simulink model "modified_splitter_IEcontrol"  (R2020a)
settings: Solver=VariableStepAuto  StartTime=0.0  StopTime=10.0  RelTol=1e-3
model workspace (MATLAB code in the model file):
  | v_M_exhale = 490; % cmH2O (PEEP)
  | v_M_inhale = 1471; % (PIP)
  | R_M = 0; %
  | 
  | R_V1 = 5670; % cmH2O/L/s
  | R_V2 = 5670;
  | R_I1 = 5670; % tube length = 1.8 ms
  | R_I2 = 5670;
  | R_EV1 = 0;
  | R_EV2 = 0;
  | 
  | R_L1 = 196133;
  | R_L2 = 196133;
  | C_L1 = 5.50647e-7; % L/cmH2O
  | C_L2 = 5.50647e-7;
  | R_ETT1 = 784000;
  | R_ETT2 = 784000;
  | 
  | % === artificial patients (bags)s ====
  | R_aL1 = 196133;
  | R_aL2 = 196133;
  | C_aL1 = 5.50647e-7;
  | C_aL2 = 5.50647e-7;
  | % =======
  | 
  | R_E1 = 5670;
  | R_E2 = 5670;
  | R_O = 0;
  | 
  | RR = 15;
  | I = 1;
  | E = 2;
  | IE_ratio = I/ E;
libraries: fl_lib x37, nesl_utility x14
settings Model: Creator=jsolislemus  LastModifiedBy=jsolislemus

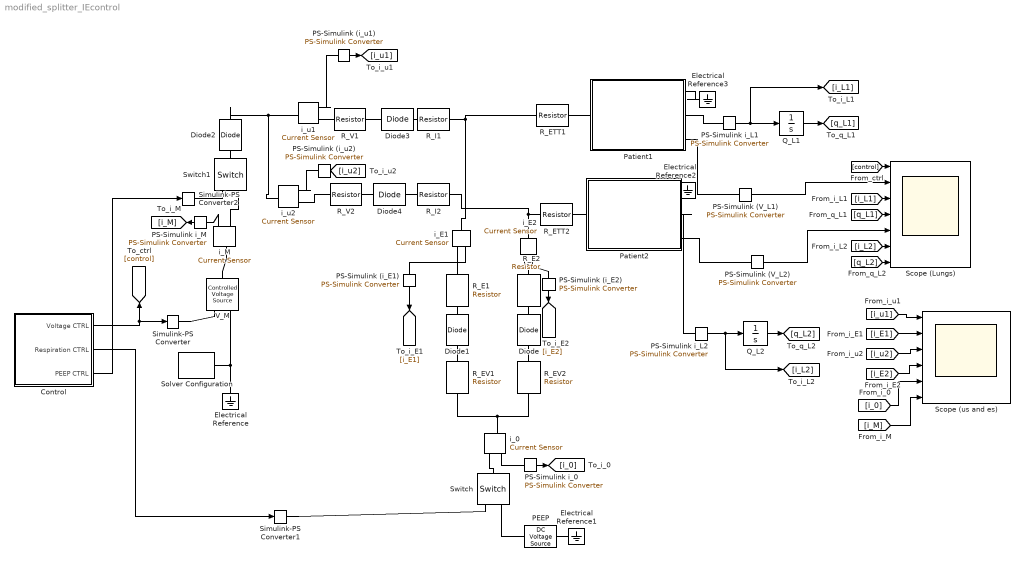
== system modified_splitter_IEcontrol ==
  Control : Subsystem
  Diode{,1..4} (5 alike) : fl_lib/Electrical/Electrical Elements/Diode  Vf=0.6 V  Ron=0.3 Ohm  Goff=1e-8 1/Ohm  i_specify=off  i_priority=None  i=0 A  i_nominal_specify=off  i_nominal_unit=A  i_nominal_value=1  v_specify=off  v_priority=None  v=0 V  v_nominal_specify=off  v_nominal_unit=V  v_nominal_value=1
  Electrical Reference{,1..3} (4 alike) : fl_lib/Electrical/Electrical Elements/Electrical Reference
  PEEP : fl_lib/Electrical/Electrical Sources/DC Voltage Source  v0=v_M_exhale V
  PS-Simulink (V_L1) : nesl_utility/PS-Simulink Converter  PhysicalDomain=network_engine_domain  SubClassName=ps_output  LeftPortType=input  RightPortType=output  PseudoPeriodic=off  Frequencies=[]  Unit=inherit  AffineConversion=off
  PS-Simulink (V_L2) : nesl_utility/PS-Simulink Converter  PhysicalDomain=network_engine_domain  SubClassName=ps_output  LeftPortType=input  RightPortType=output  PseudoPeriodic=off  Frequencies=[]  Unit=inherit  AffineConversion=off
  PS-Simulink (i_E1) : nesl_utility/PS-Simulink Converter  PhysicalDomain=network_engine_domain  SubClassName=ps_output  LeftPortType=input  RightPortType=output  PseudoPeriodic=off  Frequencies=[]  Unit=inherit  AffineConversion=off
  PS-Simulink (i_E2) : nesl_utility/PS-Simulink Converter  PhysicalDomain=network_engine_domain  SubClassName=ps_output  LeftPortType=input  RightPortType=output  PseudoPeriodic=off  Frequencies=[]  Unit=inherit  AffineConversion=off
  PS-Simulink (i_u1) : nesl_utility/PS-Simulink Converter  PhysicalDomain=network_engine_domain  SubClassName=ps_output  LeftPortType=input  RightPortType=output  PseudoPeriodic=off  Frequencies=[]  Unit=inherit  AffineConversion=off
  PS-Simulink (i_u2) : nesl_utility/PS-Simulink Converter  PhysicalDomain=network_engine_domain  SubClassName=ps_output  LeftPortType=input  RightPortType=output  PseudoPeriodic=off  Frequencies=[]  Unit=inherit  AffineConversion=off
  PS-Simulink i_0 : nesl_utility/PS-Simulink Converter  PhysicalDomain=network_engine_domain  SubClassName=ps_output  LeftPortType=input  RightPortType=output  PseudoPeriodic=off  Frequencies=[]  Unit=inherit  AffineConversion=off
  PS-Simulink i_L1 : nesl_utility/PS-Simulink Converter  PhysicalDomain=network_engine_domain  SubClassName=ps_output  LeftPortType=input  RightPortType=output  PseudoPeriodic=off  Frequencies=[]  Unit=inherit  AffineConversion=off
  PS-Simulink i_L2 : nesl_utility/PS-Simulink Converter  PhysicalDomain=network_engine_domain  SubClassName=ps_output  LeftPortType=input  RightPortType=output  PseudoPeriodic=off  Frequencies=[]  Unit=inherit  AffineConversion=off
  PS-Simulink i_M : nesl_utility/PS-Simulink Converter  PhysicalDomain=network_engine_domain  SubClassName=ps_output  LeftPortType=input  RightPortType=output  PseudoPeriodic=off  Frequencies=[]  Unit=inherit  AffineConversion=off
  Patient1 : Subsystem
  Patient2 : Subsystem
  Q_L1 : Integrator
  Q_L2 : Integrator
  R_E1 : fl_lib/Electrical/Electrical Elements/Resistor  R=R_E1 Ohm  i_specify=off  i_priority=None  i=0 A  i_nominal_specify=off  i_nominal_unit=A  i_nominal_value=1  v_specify=off  v_priority=None  v=0 V  v_nominal_specify=off  v_nominal_unit=V  v_nominal_value=1
  R_E2 : fl_lib/Electrical/Electrical Elements/Resistor  R=R_E2 Ohm  i_specify=off  i_priority=None  i=0 A  i_nominal_specify=off  i_nominal_unit=A  i_nominal_value=1  v_specify=off  v_priority=None  v=0 V  v_nominal_specify=off  v_nominal_unit=V  v_nominal_value=1
  R_ETT1 : fl_lib/Electrical/Electrical Elements/Resistor  R=R_ETT1 Ohm  i_specify=off  i_priority=None  i=0 A  i_nominal_specify=off  i_nominal_unit=A  i_nominal_value=1  v_specify=off  v_priority=None  v=0 V  v_nominal_specify=off  v_nominal_unit=V  v_nominal_value=1
  R_ETT2 : fl_lib/Electrical/Electrical Elements/Resistor  R=R_ETT2 Ohm  i_specify=off  i_priority=None  i=0 A  i_nominal_specify=off  i_nominal_unit=A  i_nominal_value=1  v_specify=off  v_priority=None  v=0 V  v_nominal_specify=off  v_nominal_unit=V  v_nominal_value=1
  R_EV1 : fl_lib/Electrical/Electrical Elements/Resistor  R=R_EV1 Ohm  i_specify=off  i_priority=None  i=0 A  i_nominal_specify=off  i_nominal_unit=A  i_nominal_value=1  v_specify=off  v_priority=None  v=0 V  v_nominal_specify=off  v_nominal_unit=V  v_nominal_value=1
  R_EV2 : fl_lib/Electrical/Electrical Elements/Resistor  R=R_EV2 Ohm  i_specify=off  i_priority=None  i=0 A  i_nominal_specify=off  i_nominal_unit=A  i_nominal_value=1  v_specify=off  v_priority=None  v=0 V  v_nominal_specify=off  v_nominal_unit=V  v_nominal_value=1
  R_I1 : fl_lib/Electrical/Electrical Elements/Resistor  R=R_I1 Ohm  i_specify=off  i_priority=None  i=0 A  i_nominal_specify=off  i_nominal_unit=A  i_nominal_value=1  v_specify=off  v_priority=None  v=0 V  v_nominal_specify=off  v_nominal_unit=V  v_nominal_value=1
  R_I2 : fl_lib/Electrical/Electrical Elements/Resistor  R=R_I2 Ohm  i_specify=off  i_priority=None  i=0 A  i_nominal_specify=off  i_nominal_unit=A  i_nominal_value=1  v_specify=off  v_priority=None  v=0 V  v_nominal_specify=off  v_nominal_unit=V  v_nominal_value=1
  R_V1 : fl_lib/Electrical/Electrical Elements/Resistor  R=R_V1 Ohm  i_specify=off  i_priority=None  i=0 A  i_nominal_specify=off  i_nominal_unit=A  i_nominal_value=1  v_specify=off  v_priority=None  v=0 V  v_nominal_specify=off  v_nominal_unit=V  v_nominal_value=1
  R_V2 : fl_lib/Electrical/Electrical Elements/Resistor  R=R_V2 Ohm  i_specify=off  i_priority=None  i=0 A  i_nominal_specify=off  i_nominal_unit=A  i_nominal_value=1  v_specify=off  v_priority=None  v=0 V  v_nominal_specify=off  v_nominal_unit=V  v_nominal_value=1
  Scope (Lungs) : Scope  NumInputPorts=7
  Scope (us and es) : Scope  NumInputPorts=6
  Simulink-PS Converter : nesl_utility/Simulink-PS Converter  PhysicalDomain=network_engine_domain  SubClassName=ps_input  LeftPortType=input  RightPortType=output  PseudoPeriodic=off  Frequencies=[]  NoiseDistribution=none  NoiseParameters=[]  Unit=1  AffineConversion=off  FilteringAndDerivatives=provide  SimscapeFilterOrder=1  InputFilterTimeConstant=0.001  UdotUserProvided=0
  Simulink-PS Converter1 : nesl_utility/Simulink-PS Converter  PhysicalDomain=network_engine_domain  SubClassName=ps_input  LeftPortType=input  RightPortType=output  PseudoPeriodic=off  Frequencies=[]  NoiseDistribution=none  NoiseParameters=[]  Unit=1  AffineConversion=off  FilteringAndDerivatives=provide  SimscapeFilterOrder=1  InputFilterTimeConstant=0.001  UdotUserProvided=0
  Simulink-PS Converter2 : nesl_utility/Simulink-PS Converter  PhysicalDomain=network_engine_domain  SubClassName=ps_input  LeftPortType=input  RightPortType=output  PseudoPeriodic=off  Frequencies=[]  NoiseDistribution=none  NoiseParameters=[]  Unit=1  AffineConversion=off  FilteringAndDerivatives=provide  SimscapeFilterOrder=1  InputFilterTimeConstant=0.001  UdotUserProvided=0
  Solver Configuration : nesl_utility/Solver Configuration  PhysicalDomain=network_engine_domain  SubClassName=solver  LeftPortType=input  RightPortType=generic  Tones=[]  Harmonics=[]  SimulateNoise=off  Profile=off  UseLocalSampling=off  EnableSwitchedLinearOptims=on  FrequencyDomain=off  UseCCode=off  RelTol=0.001  AbsTol=1e-06  MinStep=1e-09  ToWorkspace=off  RevertToSquareIcSolve=off  NumHomotopyIterations=100  PhasorMode=off  PhasorModeNumHarmonics=1  DoDC=off  ResidualTolerance=1e-09  UseLocalSolver=off  LocalSolverChoice=NE_BACKWARD_EULER_ADVANCER  LocalSolverSampleTime=0.001  DoFixedCost=off  MaxNonlinIter=3  MaxModeIter=2  LinearAlgebra=auto  EquationFormulation=NE_TIME_EF  DelaysMemoryBudget=1024  AutomaticFiltering=on  FilteringTimeConstant=0.001  PartitionStorageMethod=AS_NEEDED  PartitionMemoryBudget=1024  PartitionMethod=ROBUST
  Switch : fl_lib/Electrical/Electrical Elements/Switch  R_closed=0.01 Ohm  G_open=1e-8 1/Ohm  Threshold=0.5  i_specify=off  i_priority=None  i=0 A  i_nominal_specify=off  i_nominal_unit=A  i_nominal_value=1  v_specify=off  v_priority=None  v=0 V  v_nominal_specify=off  v_nominal_unit=V  v_nominal_value=1
  Switch1 : fl_lib/Electrical/Electrical Elements/Switch  R_closed=0.01 Ohm  G_open=1e-8 1/Ohm  Threshold=0.5  i_specify=off  i_priority=None  i=0 A  i_nominal_specify=off  i_nominal_unit=A  i_nominal_value=1  v_specify=off  v_priority=None  v=0 V  v_nominal_specify=off  v_nominal_unit=V  v_nominal_value=1
  V_M : fl_lib/Electrical/Electrical Sources/Controlled Voltage Source
  i_0 : fl_lib/Electrical/Electrical Sensors/Current Sensor
  i_E1 : fl_lib/Electrical/Electrical Sensors/Current Sensor
  i_E2 : fl_lib/Electrical/Electrical Sensors/Current Sensor
  i_M : fl_lib/Electrical/Electrical Sensors/Current Sensor
  i_u1 : fl_lib/Electrical/Electrical Sensors/Current Sensor
  i_u2 : fl_lib/Electrical/Electrical Sensors/Current Sensor
  wires:
  PS-Simulink i_L1/1 -> [i_L1], Q_L1/1
  PS-Simulink i_L2/1 -> [i_L2], Q_L2/1
  Q_L1/1 -> [q_L1]
  Q_L2/1 -> [q_L2]
  PS-Simulink (i_u1)/1 -> [i_u1]
  [i_u1] -> Scope (us and es)/1
  [i_u2] -> Scope (us and es)/3
  PS-Simulink (i_u2)/1 -> [i_u2]
  [i_E1] -> Scope (us and es)/2
  [i_E2] -> Scope (us and es)/4
  PS-Simulink (i_E2)/1 -> [i_E2]
  [i_0] -> Scope (us and es)/5
  PS-Simulink i_0/1 -> [i_0]
  PS-Simulink i_M/1 -> [i_M]
  [i_M] -> Scope (us and es)/6
  PS-Simulink (i_E1)/1 -> [i_E1]
  [control] -> Scope (Lungs)/1
  [q_L2] -> Scope (Lungs)/7
  [i_L2] -> Scope (Lungs)/6
  [q_L1] -> Scope (Lungs)/4
  PS-Simulink (V_L1)/1 -> Scope (Lungs)/2
  PS-Simulink (V_L2)/1 -> Scope (Lungs)/5
  [i_L1] -> Scope (Lungs)/3
  Control/1(Voltage CTRL) -> [control], Simulink-PS Converter/1
  Control/2(Respiration CTRL) -> Simulink-PS Converter1/1
  Control/3(PEEP CTRL) -> Simulink-PS Converter2/1
  connections:
  Simulink-PS Converter/RConn1 -- V_M/RConn1
  V_M/RConn2 -- Solver Configuration/RConn1 -- Electrical Reference/LConn1
  i_u1/LConn1 -- Diode2/RConn1 -- i_u2/LConn1
  R_ETT2/LConn1 -- R_I2/RConn1 -- i_E2/LConn1
  Simulink-PS Converter1/RConn1 -- Switch/RConn1
  i_u1/RConn2 -- R_V1/LConn1
  i_u2/RConn2 -- R_V2/LConn1
  i_E2/RConn2 -- R_E2/LConn1
  i_M/LConn1 -- V_M/LConn1
  i_0/RConn2 -- Switch/LConn1
  i_u1/RConn1 -- PS-Simulink (i_u1)/LConn1
  i_u2/RConn1 -- PS-Simulink (i_u2)/LConn1
  i_0/RConn1 -- PS-Simulink i_0/LConn1
  i_E2/RConn1 -- PS-Simulink (i_E2)/LConn1
  i_E1/RConn1 -- PS-Simulink (i_E1)/LConn1
  i_M/RConn1 -- PS-Simulink i_M/LConn1
  Electrical Reference3/LConn1 -- Patient1/RConn1
  Patient1/RConn2 -- PS-Simulink i_L1/LConn1
  Patient1/RConn3 -- PS-Simulink (V_L1)/LConn1
  Electrical Reference2/LConn1 -- Patient2/RConn1
  Patient2/RConn3 -- PS-Simulink (V_L2)/LConn1
  Patient2/RConn2 -- PS-Simulink i_L2/LConn1
  R_E1/LConn1 -- i_E1/RConn2
  R_ETT1/RConn1 -- Patient1/LConn1
  R_ETT1/LConn1 -- i_E1/LConn1 -- R_I1/RConn1
  R_ETT2/RConn1 -- Patient2/LConn1
  Diode/LConn1 -- R_E2/RConn1
  Switch1/LConn1 -- Diode2/LConn1
  Switch1/RConn2 -- i_M/RConn2
  Simulink-PS Converter2/RConn1 -- Switch1/RConn1
  PEEP/RConn1 -- Electrical Reference1/LConn1
  Switch/RConn2 -- PEEP/LConn1
  Diode1/LConn1 -- R_E1/RConn1
  Diode3/LConn1 -- R_V1/RConn1
  Diode3/RConn1 -- R_I1/LConn1
  Diode4/LConn1 -- R_V2/RConn1
  Diode4/RConn1 -- R_I2/LConn1
  R_EV1/LConn1 -- Diode1/RConn1
  R_EV2/LConn1 -- Diode/RConn1
  R_EV1/RConn1 -- R_EV2/RConn1 -- i_0/LConn1

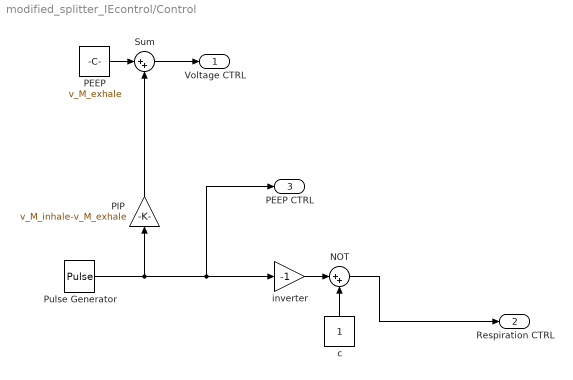
== system modified_splitter_IEcontrol/Control ==
  NOT : Sum  Inputs=|++
  PEEP : Constant  Value=v_M_exhale
  PIP : Gain  Gain=v_M_inhale-v_M_exhale
  Pulse Generator : DiscretePulseGenerator  PulseType=Time based  Period=60 / RR  PulseWidth=IE_ratio/(IE_ratio+1)*100
  Sum : Sum  Inputs=|++
  c : Constant
  inverter : Gain  Gain=-1
  Voltage CTRL : Outport
  Respiration CTRL : Outport  Port=2
  PEEP CTRL : Outport  Port=3
  wires:
  NOT/1 -> Respiration CTRL/1
  Pulse Generator/1 -> PEEP CTRL/1, inverter/1, PIP/1
  inverter/1 -> NOT/1
  Sum/1 -> Voltage CTRL/1
  PEEP/1 -> Sum/1
  PIP/1 -> Sum/2
  c/1 -> NOT/2

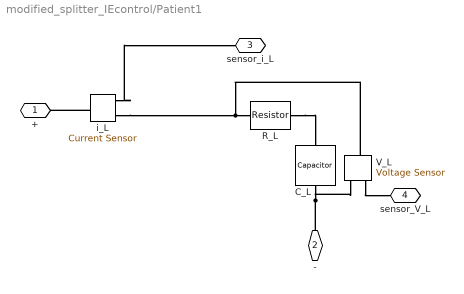
== system modified_splitter_IEcontrol/Patient1 ==
  C_L : fl_lib/Electrical/Electrical Elements/Capacitor  c=C_L1 F  r=1e-6 Ohm  g=0 1/Ohm  i_specify=off  i_priority=None  i=0 A  i_nominal_specify=off  i_nominal_unit=A  i_nominal_value=1  v_specify=off  v_priority=None  v=0 V  v_nominal_specify=off  v_nominal_unit=V  v_nominal_value=1  vc_specify=off  vc_priority=High  vc=0 V  vc_nominal_specify=off  vc_nominal_unit=V  vc_nominal_value=1
  R_L : fl_lib/Electrical/Electrical Elements/Resistor  R=R_L1 Ohm  i_specify=off  i_priority=None  i=0 A  i_nominal_specify=off  i_nominal_unit=A  i_nominal_value=1  v_specify=off  v_priority=None  v=0 V  v_nominal_specify=off  v_nominal_unit=V  v_nominal_value=1
  V_L : fl_lib/Electrical/Electrical Sensors/Voltage Sensor
  i_L : fl_lib/Electrical/Electrical Sensors/Current Sensor
  + : PMIOPort  Side=Left
  - : PMIOPort  Port=2  Side=Right
  sensor_i_L : PMIOPort  Port=3  Side=Right
  sensor_V_L : PMIOPort  Port=4  Side=Right
  connections:
  i_L/LConn1 -- +/RConn1
  C_L/RConn1 -- V_L/RConn2 -- -/RConn1
  i_L/RConn1 -- sensor_i_L/RConn1
  V_L/RConn1 -- sensor_V_L/RConn1
  R_L/RConn1 -- C_L/LConn1
  R_L/LConn1 -- i_L/RConn2 -- V_L/LConn1

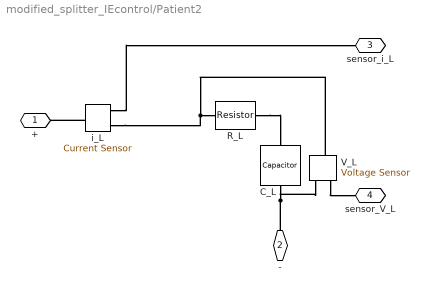
== system modified_splitter_IEcontrol/Patient2 ==
  C_L : fl_lib/Electrical/Electrical Elements/Capacitor  c=C_L2 F  r=1e-6 Ohm  g=0 1/Ohm  i_specify=off  i_priority=None  i=0 A  i_nominal_specify=off  i_nominal_unit=A  i_nominal_value=1  v_specify=off  v_priority=None  v=0 V  v_nominal_specify=off  v_nominal_unit=V  v_nominal_value=1  vc_specify=off  vc_priority=High  vc=0 V  vc_nominal_specify=off  vc_nominal_unit=V  vc_nominal_value=1
  R_L : fl_lib/Electrical/Electrical Elements/Resistor  R=R_L2 Ohm  i_specify=off  i_priority=None  i=0 A  i_nominal_specify=off  i_nominal_unit=A  i_nominal_value=1  v_specify=off  v_priority=None  v=0 V  v_nominal_specify=off  v_nominal_unit=V  v_nominal_value=1
  V_L : fl_lib/Electrical/Electrical Sensors/Voltage Sensor
  i_L : fl_lib/Electrical/Electrical Sensors/Current Sensor
  + : PMIOPort  Side=Left
  - : PMIOPort  Port=2  Side=Right
  sensor_i_L : PMIOPort  Port=3  Side=Right
  sensor_V_L : PMIOPort  Port=4  Side=Right
  connections:
  i_L/LConn1 -- +/RConn1
  V_L/RConn2 -- C_L/RConn1 -- -/RConn1
  i_L/RConn1 -- sensor_i_L/RConn1
  V_L/RConn1 -- sensor_V_L/RConn1
  R_L/RConn1 -- C_L/LConn1
  V_L/LConn1 -- i_L/RConn2 -- R_L/LConn1
